simulink model "anw_pid1"  (Simulink 4.00)
settings: Solver=ode45  StartTime=0.0  StopTime=10  RelTol=1e-3
values from neighbouring files (symbols this model uses):
  b = 1    [anw_pid_1.m]    (also in mehrw_4.m = my_system1.b; mehrw_5.m = my_system1.b)
  K = 5    [anw_pid_1.m]
  N = 5    [anw_pid_1.m]    (also in inv_switch_1.m = 200)
  Td = 80    [anw_pid_1.m]
  Ti = 0.05    [anw_pid_1.m]
  Tt = 1    [anw_pid_1.m]
settings Model: LastModifiedBy=Administrator  Refine=5  BlockReductionOpt=off

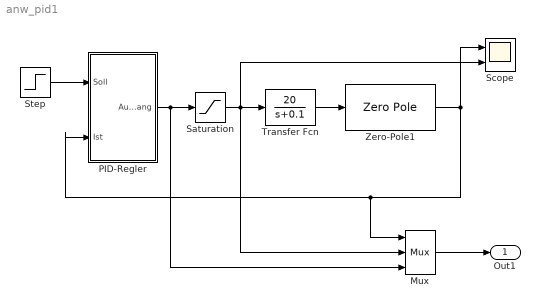
== system anw_pid1 ==
  Mux : Mux  Inputs=3
      settings: DisplayOption=none
  PID-Regler : Subsystem
      settings: RTWFcnNameOpts=Auto  RTWFileNameOpts=Auto
  Saturation : Saturate  UpperLimit=1  LowerLimit=-1  LinearizeAsGain=on
  Scope : Scope  NumInputPorts=2
      settings: TimeRange=auto  YMin=-5~-5  YMax=5~5  SaveToWorkspace=off  SaveName=ScopeData  LimitDataPoints=on  MaxDataPoints=5000
  Step : Step  Time=0  Before=0  After=1  SampleTime=0
  Transfer Fcn : TransferFcn  Numerator=[20]  Denominator=[1 0.1]  Realization=auto  AbsoluteTolerance=auto
  Zero-Pole1 : ZeroPole  Zeros=[-0.5]  Poles=[-1 -5]  Gain=[1]  AbsoluteTolerance=auto
  Out1 : Outport  Port=1
  wires:
  Step/1 -> PID-Regler/1(Soll)
  PID-Regler/1(Ausgang) -> Saturation/1, Mux/3
  Saturation/1 -> Transfer Fcn/1, Scope/2, Mux/2
  Transfer Fcn/1 -> Zero-Pole1/1
  Zero-Pole1/1 -> Scope/1, PID-Regler/2(Ist), Mux/1
  Mux/1 -> Out1/1

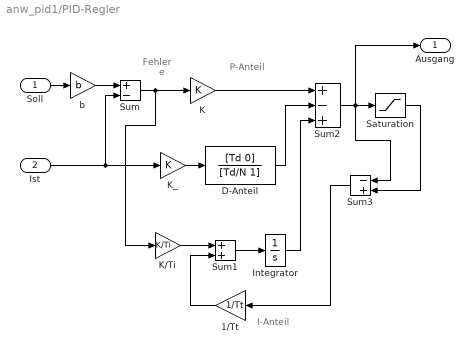
== system anw_pid1/PID-Regler ==
  note: I-Anteil
  note: e
  note: Fehler
  note: P-Anteil
  Soll : Inport  Port=1
  Ist : Inport  Port=2
  1/Tt : Gain  Orientation=left  Gain=1/Tt  Multiplication=Element-wise(K.*u)  SaturateOnIntegerOverflow=on
  "D-Anteil " : TransferFcn  Numerator=[Td 0]  Denominator=[Td/N 1]  Realization=auto  AbsoluteTolerance=auto
  Integrator : Integrator  ExternalReset=none  InitialConditionSource=internal  InitialCondition=0  LimitOutput=off  UpperSaturationLimit=inf  LowerSaturationLimit=-inf  ShowSaturationPort=off  ShowStatePort=off  AbsoluteTolerance=auto
  K : Gain  Gain=K  Multiplication=Element-wise(K.*u)  SaturateOnIntegerOverflow=on
  K/Ti : Gain  Gain=K/Ti  Multiplication=Element-wise(K.*u)  SaturateOnIntegerOverflow=on
  K_ : Gain  Gain=K  Multiplication=Element-wise(K.*u)  SaturateOnIntegerOverflow=on
  Saturation : Saturate  UpperLimit=1  LowerLimit=-1  LinearizeAsGain=on
  Sum : Sum  Inputs=+-  SaturateOnIntegerOverflow=on
  Sum1 : Sum  Inputs=++  SaturateOnIntegerOverflow=on
  Sum2 : Sum  Inputs=+-+  SaturateOnIntegerOverflow=on
  Sum3 : Sum  Orientation=left  Inputs=-+  SaturateOnIntegerOverflow=on
  b : Gain  Gain=b  Multiplication=Element-wise(K.*u)  SaturateOnIntegerOverflow=on
  Ausgang : Outport  Port=1
  wires:
  Sum2/1 -> Saturation/1, Sum3/1, Ausgang/1
  Saturation/1 -> Sum3/2
  K/1 -> Sum2/1
  b/1 -> Sum/1
  K_/1 -> "D-Anteil "/1
  "D-Anteil "/1 -> Sum2/2
  Integrator/1 -> Sum2/3
  Sum1/1 -> Integrator/1
  K/Ti/1 -> Sum1/1
  Sum/1 -> K/1, K/Ti/1
  1/Tt/1 -> Sum1/2
  Sum3/1 -> 1/Tt/1
  Soll/1 -> b/1
  Ist/1 -> Sum/2, K_/1
